simulink model "vertMotorSimTab"  (R2025a)
settings: Solver=FixedStepDiscrete  StartTime=0.0  StopTime=10  FixedStep=0.002  RelTol=1e-3  EnableMultiTasking=on
settings Model: ExtModeTrigDuration=10000  Creator=jellu  LastModifiedBy=Ayush_S
settings SolverCC: AlgebraicLoopSolver=TrustRegion  PositivePriorityOrder=on
settings DataIOCC: ReturnWorkspaceOutputs=off
settings OptimizationCC: LifeSpan=inf
settings DebuggingCC: UnconnectedInputMsg=warning  UnconnectedOutputMsg=warning  UnconnectedLineMsg=warning  ArithmeticOperatorsInVariantConditions=warning
settings ModelReferenceCC: EnableRefExpFcnMdlSchedulingChecks=on
settings SFSimCC: SimUseLocalCustomCode=off  CustomCodeUndefinedFunction=UseInterfaceOnly
settings RTWCC: SystemTargetFile=quarc_win64.tlc  TemplateMakefile=quarc_default_tmf  RTWUseLocalCustomCode=off  GPUComputeCapability=3.5  Description=QUARC Win64 Target
settings CodeAppCC: StateflowObjectComments=on
settings STFCustomTargetCC: SystemTargetFile=quarc_win64.tlc  TargetPreCompLibLocation=C:\PROGRA~3\QUARC\lib\2016a\win64\release  TargetLangStandard=C99 (ISO)  MultiwordLength=2048.0  DynamicStringBufferSize=256.0  ConcurrentExecutionCompliant=on  StopOnOverrun=off  DownloadToTarget=on  Debug=off
settings GRTTargetCC: ExtMode=on  ExtModeMexFile=quarc_comm  TargetPreCompLibLocation=C:\PROGRA~3\QUARC\lib\2016a\win64\release  ParMdlRefBuildCompliant=off  CompOptLevelCompliant=off  CombineOutputUpdateFcns=off  MatFileLogging=off  CPPClassGenCompliant=off  GRTInterface=on  UseToolchainInfoCompliant=off
settings ConfigComp: CovMetricSettings=dswe

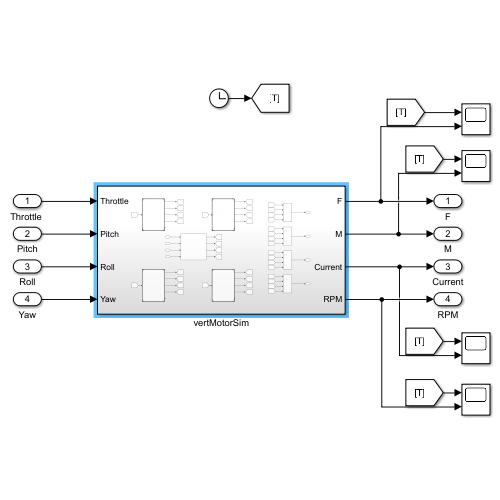
[thumbnail: Simulink's stored preview of the top-level diagram]
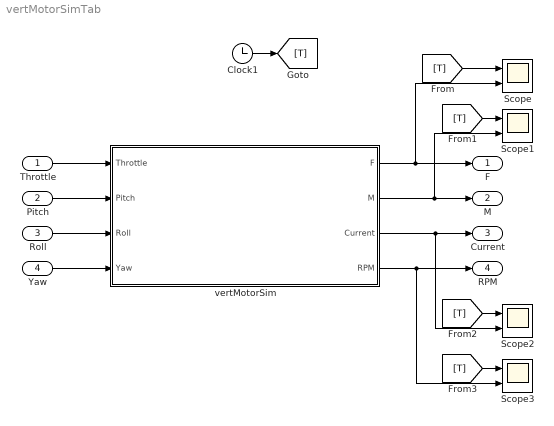
== system vertMotorSimTab ==
  "Throttle " : Inport
  Pitch : Inport  Port=2
  Roll : Inport  Port=3
  Yaw : Inport  Port=4
  Clock1 : Clock
  Scope{,1..3} (4 alike) : Scope  NumInputPorts=2
      Scope settings: ActiveDisplayYMinimum=-1  ActiveDisplayYMaximum=1
      Scope1 settings: ActiveDisplayYMinimum=-1  ActiveDisplayYMaximum=1
      Scope2 settings: ActiveDisplayYMinimum=-1  ActiveDisplayYMaximum=1  DataLoggingVariableName=ScopeData2
      Scope3 settings: ActiveDisplayYMinimum=-1  ActiveDisplayYMaximum=1  DataLoggingVariableName=ScopeData3
  vertMotorSim : Subsystem
  F : Outport
  M : Outport  Port=2
  Current : Outport  Port=3
  RPM : Outport  Port=4
  wires:
  "Throttle "/1 -> vertMotorSim/1(Throttle)
  vertMotorSim/1(F) -> Scope/2, F/1
  vertMotorSim/2(M) -> Scope1/2, M/1
  vertMotorSim/3(Current) -> Scope2/2, Current/1
  vertMotorSim/4(RPM) -> Scope3/2, RPM/1
  Pitch/1 -> vertMotorSim/2(Pitch)
  Roll/1 -> vertMotorSim/3(Roll)
  Yaw/1 -> vertMotorSim/4(Yaw)
  [T] -> Scope/1
  Clock1/1 -> [T]
  [T] -> Scope1/1
  [T] -> Scope2/1
  [T] -> Scope3/1

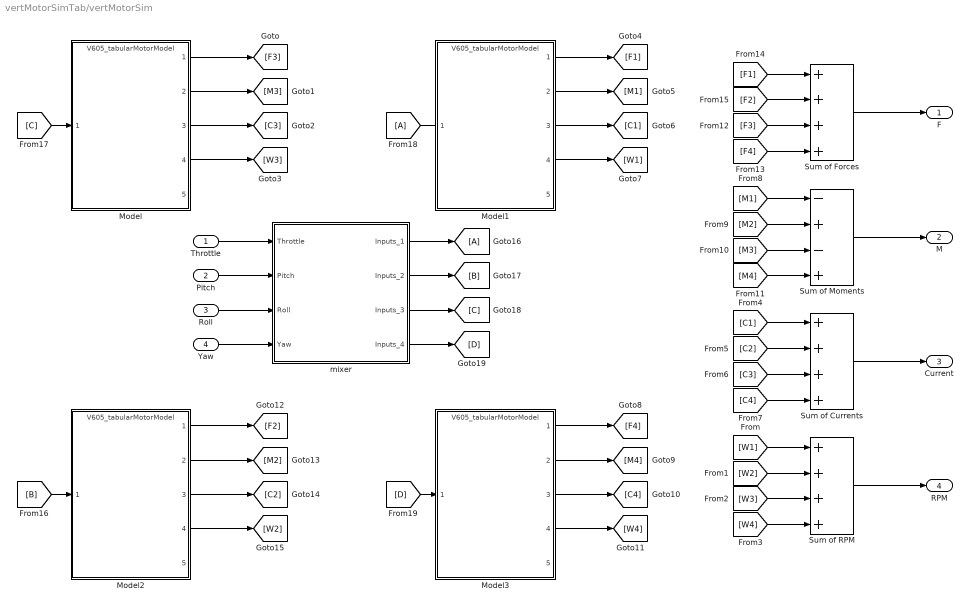
== system vertMotorSimTab/vertMotorSim ==
  Throttle : Inport
  Pitch : Inport  Port=2
  Roll : Inport  Port=3
  Yaw : Inport  Port=4
  From18 : From
  Goto16 : Goto
  Model{,1..3} (4 alike) : ModelReference  ModelNameDialog=V605_tabularMotorModel.slx  SimulationMode=Normal  ModelReferenceVersion=3.0
  Sum of Currents : Sum  Inputs=++++
  Sum of Forces : Sum  Inputs=++++
  Sum of Moments : Sum  Inputs=-+-+
  Sum of RPM : Sum  Inputs=++++
  mixer : Subsystem
  F : Outport
  M : Outport  Port=2
  Current : Outport  Port=3
  RPM : Outport  Port=4
  wires:
  Sum of RPM/1 -> RPM/1
  Sum of Currents/1 -> Current/1
  Sum of Moments/1 -> M/1
  Sum of Forces/1 -> F/1
  Throttle/1 -> mixer/1(Throttle)
  Model/1 -> [F3]
  Model/2 -> [M3]
  Model/3 -> [C3]
  Model/4 -> [W3]
  [W1] -> Sum of RPM/1
  [W2] -> Sum of RPM/2
  [W3] -> Sum of RPM/3
  [W4] -> Sum of RPM/4
  [C1] -> Sum of Currents/1
  [C2] -> Sum of Currents/2
  [C3] -> Sum of Currents/3
  [C4] -> Sum of Currents/4
  Model1/1 -> [F1]
  Model1/3 -> [C1]
  Model1/2 -> [M1]
  Model1/4 -> [W1]
  Model3/3 -> [C4]
  Model3/2 -> [M4]
  Model3/4 -> [W4]
  Model2/2 -> [M2]
  Model2/3 -> [C2]
  Model3/1 -> [F4]
  Model2/4 -> [W2]
  Model2/1 -> [F2]
  [M1] -> Sum of Moments/1
  [M2] -> Sum of Moments/2
  [M3] -> Sum of Moments/3
  [M4] -> Sum of Moments/4
  [F1] -> Sum of Forces/1
  [F2] -> Sum of Forces/2
  [F3] -> Sum of Forces/3
  [F4] -> Sum of Forces/4
  Pitch/1 -> mixer/2(Pitch)
  Roll/1 -> mixer/3(Roll)
  Yaw/1 -> mixer/4(Yaw)
  mixer/1(" Inputs_1") -> Goto16/1
  mixer/2(Inputs_2) -> [B]
  [B] -> Model2/1
  mixer/3(Inputs_3) -> [C]
  [C] -> Model/1
  From18/1 -> ?
  [D] -> Model3/1
  mixer/4(Inputs_4) -> [D]

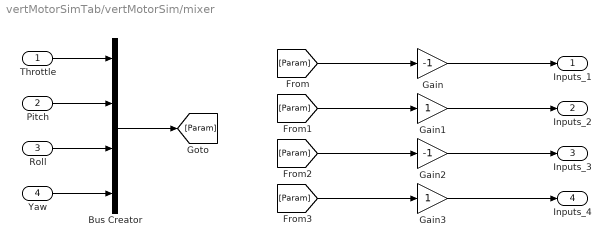
== system vertMotorSimTab/vertMotorSim/mixer ==
  Throttle : Inport
  Pitch : Inport  Port=2
  Roll : Inport  Port=3
  Yaw : Inport  Port=4
  Bus Creator : BusCreator  Inputs=4
  Gain : Gain  Gain=-1
  Gain1 : Gain
  Gain2 : Gain  Gain=-1
  Gain3 : Gain
  " Inputs_1" : Outport
  Inputs_2 : Outport  Port=2
  Inputs_3 : Outport  Port=3
  Inputs_4 : Outport  Port=4
  wires:
  Throttle/1 -> Bus Creator/1
  Pitch/1 -> Bus Creator/2
  Roll/1 -> Bus Creator/3
  Yaw/1 -> Bus Creator/4
  Bus Creator/1 -> [Param]
  Gain/1 -> " Inputs_1"/1
  [Param] -> Gain/1
  [Param] -> Gain1/1
  Gain1/1 -> Inputs_2/1
  [Param] -> Gain2/1
  Gain2/1 -> Inputs_3/1
  [Param] -> Gain3/1
  Gain3/1 -> Inputs_4/1
